simulink model "case9"  (R2024b)
settings: Solver=FixedStepAuto  StartTime=0  StopTime=1  FixedStep=1e-7  RelTol=1e-3
values from neighbouring files (symbols this model uses):
  SG_D_1_D = 0.01056    [IEEE9_case_parameters.m]    (also in case1_parameters.m; case2_parameters.m; case3_parameters.m; case4_parameters.m)
  SG_D_1_EnableSaturation = 0    [IEEE9_case_parameters.m]    (also in case1_parameters.m; case2_parameters.m; case3_parameters.m; case4_parameters.m)
  SG_D_1_f0 = 60    [IEEE9_case_parameters.m]    (also in case1_parameters.m; case2_parameters.m; case3_parameters.m; case4_parameters.m)
  SG_D_1_H = 7.5    [IEEE9_case_parameters.m]    (also in case1_parameters.m; case2_parameters.m; case3_parameters.m; case4_parameters.m)
  SG_D_1_K_A = 20    [IEEE9_case_parameters.m]    (also in case1_parameters.m; case2_parameters.m; case3_parameters.m; case4_parameters.m)
  SG_D_1_K_E = 1.000000e+1    (= 10)    [IEEE9_case_parameters.m]    (also in case1_parameters.m; case2_parameters.m; case3_parameters.m; case4_parameters.m)
  SG_D_1_K_F = 2.363    [IEEE9_case_parameters.m]    (also in case1_parameters.m; case2_parameters.m; case3_parameters.m; case4_parameters.m)
  SG_D_1_K_s = 0.5    [IEEE9_case_parameters.m]    (also in case1_parameters.m = 5; case2_parameters.m = 5; case3_parameters.m = 5; case4_parameters.m = 5)
  SG_D_1_R_a = 0.001088    [IEEE9_case_parameters.m]    (also in case1_parameters.m; case2_parameters.m; case3_parameters.m; case4_parameters.m)
  SG_D_1_S_A = 1    [IEEE9_case_parameters.m]    (also in case1_parameters.m; case2_parameters.m; case3_parameters.m; case4_parameters.m)
  SG_D_1_S_B = 0.103    [IEEE9_case_parameters.m]    (also in case1_parameters.m; case2_parameters.m; case3_parameters.m; case4_parameters.m)
  SG_D_1_S_N = 10.659857    [IEEE9_case_parameters.m]    (also in case1_parameters.m; case2_parameters.m; case3_parameters.m; case4_parameters.m)
  SG_D_1_SpeedPara = 200    [IEEE9_case_parameters.m]    (also in case1_parameters.m; case2_parameters.m; case3_parameters.m; case4_parameters.m)
  SG_D_1_T_0 = 0.720173    [IEEE9_case_parameters.m]    (also in case1_parameters.m = 0.755522; case2_parameters.m = 0.808931; case3_parameters.m = 0.869402; case4_parameters.m = 0.729316)
  SG_D_1_T_1 = 0.3    [IEEE9_case_parameters.m]    (also in case1_parameters.m; case2_parameters.m; case3_parameters.m; case4_parameters.m)
  SG_D_1_T_2 = 0.05    [IEEE9_case_parameters.m]    (also in case1_parameters.m; case2_parameters.m; case3_parameters.m; case4_parameters.m)
  SG_D_1_T_3 = 0.02    [IEEE9_case_parameters.m]    (also in case1_parameters.m; case2_parameters.m; case3_parameters.m; case4_parameters.m)
  SG_D_1_T_4 = 0.005    [IEEE9_case_parameters.m]    (also in case1_parameters.m; case2_parameters.m; case3_parameters.m; case4_parameters.m)
  SG_D_1_T_A = 0.02    [IEEE9_case_parameters.m]    (also in case1_parameters.m; case2_parameters.m; case3_parameters.m; case4_parameters.m)
  SG_D_1_T_dd = 8.000000e+0    (= 8)    [IEEE9_case_parameters.m]    (also in case1_parameters.m; case2_parameters.m; case3_parameters.m; case4_parameters.m)
  SG_D_1_T_ddd = 0.04    [IEEE9_case_parameters.m]    (also in case1_parameters.m; case2_parameters.m; case3_parameters.m; case4_parameters.m)
  SG_D_1_T_E = 0.314    [IEEE9_case_parameters.m]    (also in case1_parameters.m; case2_parameters.m; case3_parameters.m; case4_parameters.m)
  SG_D_1_T_F = 0.35    [IEEE9_case_parameters.m]    (also in case1_parameters.m; case2_parameters.m; case3_parameters.m; case4_parameters.m)
  SG_D_1_T_qd = 0.8    [IEEE9_case_parameters.m]    (also in case1_parameters.m; case2_parameters.m; case3_parameters.m; case4_parameters.m)
  SG_D_1_T_qdd = 0.02    [IEEE9_case_parameters.m]    (also in case1_parameters.m; case2_parameters.m; case3_parameters.m; case4_parameters.m)
  SG_D_1_T_speed = 0.1    [IEEE9_case_parameters.m]    (also in case1_parameters.m = 200; case2_parameters.m = 200; case3_parameters.m = 200; case4_parameters.m = 200)
  SG_D_1_T_w = 0.5    [IEEE9_case_parameters.m]    (also in case1_parameters.m; case2_parameters.m; case3_parameters.m; case4_parameters.m)
  SG_D_1_V_ref = 1.990276    [IEEE9_case_parameters.m]    (also in case1_parameters.m = 2.042296; case2_parameters.m = 2.051388; case3_parameters.m = 2.089584; case4_parameters.m = 2.01845)
  SG_D_1_w_ref = 376.991118    [IEEE9_case_parameters.m]    (also in case1_parameters.m; case2_parameters.m; case3_parameters.m; case4_parameters.m)
  SG_D_1_wb = 6.000000e+1    (= 60)    [IEEE9_case_parameters.m]    (also in case1_parameters.m; case2_parameters.m; case3_parameters.m; case4_parameters.m)
  SG_D_1_x_d = 1.9    [IEEE9_case_parameters.m]    (also in case1_parameters.m; case2_parameters.m; case3_parameters.m; case4_parameters.m)
  SG_D_1_x_dd = 0.302    [IEEE9_case_parameters.m]    (also in case1_parameters.m; case2_parameters.m; case3_parameters.m; case4_parameters.m)
  SG_D_1_x_ddd = 0.204    [IEEE9_case_parameters.m]    (also in case1_parameters.m; case2_parameters.m; case3_parameters.m; case4_parameters.m)
  SG_D_1_x_l = 0.05    [IEEE9_case_parameters.m]    (also in case1_parameters.m; case2_parameters.m; case3_parameters.m; case4_parameters.m)
  SG_D_1_x_q = 1.3    [IEEE9_case_parameters.m]    (also in case1_parameters.m; case2_parameters.m; case3_parameters.m; case4_parameters.m)
  SG_D_1_x_qd = 0.5    [IEEE9_case_parameters.m]    (also in case1_parameters.m; case2_parameters.m; case3_parameters.m; case4_parameters.m)
  SG_D_1_x_qdd = 0.3    [IEEE9_case_parameters.m]    (also in case1_parameters.m; case2_parameters.m; case3_parameters.m; case4_parameters.m)
  SG_D_2_D = 0.02    [IEEE9_case_parameters.m]    (also in case1_parameters.m; case2_parameters.m; case3_parameters.m; case4_parameters.m)
  SG_D_2_EnableSaturation = 0    [IEEE9_case_parameters.m]    (also in case1_parameters.m; case2_parameters.m; case3_parameters.m; case4_parameters.m)
  SG_D_2_f0 = 60    [IEEE9_case_parameters.m]    (also in case1_parameters.m; case2_parameters.m; case3_parameters.m; case4_parameters.m)
  SG_D_2_H = 8.000000e+0    (= 8)    [IEEE9_case_parameters.m]    (also in case1_parameters.m; case2_parameters.m; case3_parameters.m; case4_parameters.m)
  SG_D_2_K_A = 20    [IEEE9_case_parameters.m]    (also in case1_parameters.m; case2_parameters.m; case3_parameters.m; case4_parameters.m)
  SG_D_2_K_E = 1.000000e+1    (= 10)    [IEEE9_case_parameters.m]    (also in case1_parameters.m; case2_parameters.m; case3_parameters.m; case4_parameters.m)
  SG_D_2_K_F = 2.363    [IEEE9_case_parameters.m]    (also in case1_parameters.m; case2_parameters.m; case3_parameters.m; case4_parameters.m)
  SG_D_2_K_s = 0.5    [IEEE9_case_parameters.m]    (also in case1_parameters.m = 4; case2_parameters.m = 4; case3_parameters.m = 4; case4_parameters.m = 4)
  SG_D_2_R_a = 0.001088    [IEEE9_case_parameters.m]    (also in case1_parameters.m; case2_parameters.m; case3_parameters.m; case4_parameters.m)
  SG_D_2_S_A = 1    [IEEE9_case_parameters.m]    (also in case1_parameters.m; case2_parameters.m; case3_parameters.m; case4_parameters.m)
  SG_D_2_S_B = 0.103    [IEEE9_case_parameters.m]    (also in case1_parameters.m; case2_parameters.m; case3_parameters.m; case4_parameters.m)
  SG_D_2_S_N = 10.659857    [IEEE9_case_parameters.m]    (also in case1_parameters.m; case2_parameters.m; case3_parameters.m; case4_parameters.m)
  SG_D_2_SpeedPara = 200    [IEEE9_case_parameters.m]    (also in case1_parameters.m; case2_parameters.m; case3_parameters.m; case4_parameters.m)
  SG_D_2_T_0 = 1.632913    [IEEE9_case_parameters.m]    (also in case1_parameters.m = 1.632925; case2_parameters.m = 1.632915; case3_parameters.m = 1.632914; case4_parameters.m = 1.632927)
  SG_D_2_T_1 = 0.2    [IEEE9_case_parameters.m]    (also in case1_parameters.m; case2_parameters.m; case3_parameters.m; case4_parameters.m)
  SG_D_2_T_2 = 0.05    [IEEE9_case_parameters.m]    (also in case1_parameters.m; case2_parameters.m; case3_parameters.m; case4_parameters.m)
  SG_D_2_T_3 = 0.02    [IEEE9_case_parameters.m]    (also in case1_parameters.m; case2_parameters.m; case3_parameters.m; case4_parameters.m)
  SG_D_2_T_4 = 0.005    [IEEE9_case_parameters.m]    (also in case1_parameters.m; case2_parameters.m; case3_parameters.m; case4_parameters.m)
  SG_D_2_T_A = 0.02    [IEEE9_case_parameters.m]    (also in case1_parameters.m; case2_parameters.m; case3_parameters.m; case4_parameters.m)
  SG_D_2_T_dd = 7.9    [IEEE9_case_parameters.m]    (also in case1_parameters.m; case2_parameters.m; case3_parameters.m; case4_parameters.m)
  SG_D_2_T_ddd = 0.04    [IEEE9_case_parameters.m]    (also in case1_parameters.m; case2_parameters.m; case3_parameters.m; case4_parameters.m)
  SG_D_2_T_E = 0.314    [IEEE9_case_parameters.m]    (also in case1_parameters.m; case2_parameters.m; case3_parameters.m; case4_parameters.m)
  SG_D_2_T_F = 0.35    [IEEE9_case_parameters.m]    (also in case1_parameters.m; case2_parameters.m; case3_parameters.m; case4_parameters.m)
  SG_D_2_T_qd = 0.8    [IEEE9_case_parameters.m]    (also in case1_parameters.m; case2_parameters.m; case3_parameters.m; case4_parameters.m)
  SG_D_2_T_qdd = 0.015    [IEEE9_case_parameters.m]    (also in case1_parameters.m; case2_parameters.m; case3_parameters.m; case4_parameters.m)
  SG_D_2_T_speed = 0.1    [IEEE9_case_parameters.m]    (also in case1_parameters.m = 150; case2_parameters.m = 150; case3_parameters.m = 150; case4_parameters.m = 150)
  SG_D_2_T_w = 0.35    [IEEE9_case_parameters.m]    (also in case1_parameters.m; case2_parameters.m; case3_parameters.m; case4_parameters.m)
  SG_D_2_V_ref = 2.58547    [IEEE9_case_parameters.m]    (also in case1_parameters.m = 2.597896; case2_parameters.m = 2.587136; case3_parameters.m = 2.586042; case4_parameters.m = 2.599679)
  SG_D_2_w_ref = 376.991118    [IEEE9_case_parameters.m]    (also in case1_parameters.m; case2_parameters.m; case3_parameters.m; case4_parameters.m)
  SG_D_2_wb = 6.000000e+1    (= 60)    [IEEE9_case_parameters.m]    (also in case1_parameters.m; case2_parameters.m; case3_parameters.m; case4_parameters.m)
  SG_D_2_x_d = 1.8    [IEEE9_case_parameters.m]    (also in case1_parameters.m; case2_parameters.m; case3_parameters.m; case4_parameters.m)
  SG_D_2_x_dd = 0.302    [IEEE9_case_parameters.m]    (also in case1_parameters.m; case2_parameters.m; case3_parameters.m; case4_parameters.m)
  SG_D_2_x_ddd = 0.204    [IEEE9_case_parameters.m]    (also in case1_parameters.m; case2_parameters.m; case3_parameters.m; case4_parameters.m)
  SG_D_2_x_l = 0.05    [IEEE9_case_parameters.m]    (also in case1_parameters.m; case2_parameters.m; case3_parameters.m; case4_parameters.m)
  SG_D_2_x_q = 1.25    [IEEE9_case_parameters.m]    (also in case1_parameters.m; case2_parameters.m; case3_parameters.m; case4_parameters.m)
  SG_D_2_x_qd = 0.5    [IEEE9_case_parameters.m]    (also in case1_parameters.m; case2_parameters.m; case3_parameters.m; case4_parameters.m)
  SG_D_2_x_qdd = 0.3    [IEEE9_case_parameters.m]    (also in case1_parameters.m; case2_parameters.m; case3_parameters.m; case4_parameters.m)
  SG_D_3_D = 0.02    [IEEE9_case_parameters.m]    (also in case1_parameters.m; case2_parameters.m; case3_parameters.m; case4_parameters.m)
  SG_D_3_EnableSaturation = 0    [IEEE9_case_parameters.m]    (also in case1_parameters.m; case2_parameters.m; case3_parameters.m; case4_parameters.m)
  SG_D_3_f0 = 60    [IEEE9_case_parameters.m]    (also in case1_parameters.m; case2_parameters.m; case3_parameters.m; case4_parameters.m)
  SG_D_3_H = 7.7    [IEEE9_case_parameters.m]    (also in case1_parameters.m; case2_parameters.m; case3_parameters.m; case4_parameters.m)
  SG_D_3_K_A = 20    [IEEE9_case_parameters.m]    (also in case1_parameters.m; case2_parameters.m; case3_parameters.m; case4_parameters.m)
  SG_D_3_K_E = 1.000000e+1    (= 10)    [IEEE9_case_parameters.m]    (also in case1_parameters.m; case2_parameters.m; case3_parameters.m; case4_parameters.m)
  SG_D_3_K_F = 2.363    [IEEE9_case_parameters.m]    (also in case1_parameters.m; case2_parameters.m; case3_parameters.m; case4_parameters.m)
  SG_D_3_K_s = 0.2    [IEEE9_case_parameters.m]    (also in case1_parameters.m = 2; case2_parameters.m = 2; case3_parameters.m = 2; case4_parameters.m = 2)
  SG_D_3_R_a = 0.001088    [IEEE9_case_parameters.m]    (also in case1_parameters.m; case2_parameters.m; case3_parameters.m; case4_parameters.m)
  SG_D_3_S_A = 1    [IEEE9_case_parameters.m]    (also in case1_parameters.m; case2_parameters.m; case3_parameters.m; case4_parameters.m)
  SG_D_3_S_B = 0.103    [IEEE9_case_parameters.m]    (also in case1_parameters.m; case2_parameters.m; case3_parameters.m; case4_parameters.m)
  SG_D_3_S_N = 10.659857    [IEEE9_case_parameters.m]    (also in case1_parameters.m; case2_parameters.m; case3_parameters.m; case4_parameters.m)
  SG_D_3_SpeedPara = 200    [IEEE9_case_parameters.m]    (also in case1_parameters.m; case2_parameters.m; case3_parameters.m; case4_parameters.m)
  SG_D_3_T_0 = 0.850788    [IEEE9_case_parameters.m]    (also in case1_parameters.m = 0.850786; case2_parameters.m = 0.850787; case3_parameters.m; case4_parameters.m = 0.850786)
  SG_D_3_T_1 = 0.2    [IEEE9_case_parameters.m]    (also in case1_parameters.m; case2_parameters.m; case3_parameters.m; case4_parameters.m)
  SG_D_3_T_2 = 0.05    [IEEE9_case_parameters.m]    (also in case1_parameters.m; case2_parameters.m; case3_parameters.m; case4_parameters.m)
  SG_D_3_T_3 = 0.02    [IEEE9_case_parameters.m]    (also in case1_parameters.m; case2_parameters.m; case3_parameters.m; case4_parameters.m)
  SG_D_3_T_4 = 0.005    [IEEE9_case_parameters.m]    (also in case1_parameters.m; case2_parameters.m; case3_parameters.m; case4_parameters.m)
  SG_D_3_T_A = 0.02    [IEEE9_case_parameters.m]    (also in case1_parameters.m; case2_parameters.m; case3_parameters.m; case4_parameters.m)
  SG_D_3_T_dd = 8.1    [IEEE9_case_parameters.m]    (also in case1_parameters.m; case2_parameters.m; case3_parameters.m; case4_parameters.m)
  SG_D_3_T_ddd = 0.04    [IEEE9_case_parameters.m]    (also in case1_parameters.m; case2_parameters.m; case3_parameters.m; case4_parameters.m)
  SG_D_3_T_E = 0.314    [IEEE9_case_parameters.m]    (also in case1_parameters.m; case2_parameters.m; case3_parameters.m; case4_parameters.m)
  SG_D_3_T_F = 0.35    [IEEE9_case_parameters.m]    (also in case1_parameters.m; case2_parameters.m; case3_parameters.m; case4_parameters.m)
  SG_D_3_T_qd = 0.8    [IEEE9_case_parameters.m]    (also in case1_parameters.m; case2_parameters.m; case3_parameters.m; case4_parameters.m)
  SG_D_3_T_qdd = 0.015    [IEEE9_case_parameters.m]    (also in case1_parameters.m; case2_parameters.m; case3_parameters.m; case4_parameters.m)
  SG_D_3_T_speed = 0.1    [IEEE9_case_parameters.m]    (also in case1_parameters.m = 180; case2_parameters.m = 180; case3_parameters.m = 180; case4_parameters.m = 180)
  SG_D_3_T_w = 0.4    [IEEE9_case_parameters.m]    (also in case1_parameters.m; case2_parameters.m; case3_parameters.m; case4_parameters.m)
  SG_D_3_V_ref = 1.892727    [IEEE9_case_parameters.m]    (also in case1_parameters.m = 1.906439; case2_parameters.m = 1.895535; case3_parameters.m = 1.892105; case4_parameters.m = 1.906598)
  SG_D_3_w_ref = 376.991118    [IEEE9_case_parameters.m]    (also in case1_parameters.m; case2_parameters.m; case3_parameters.m; case4_parameters.m)
  SG_D_3_wb = 6.000000e+1    (= 60)    [IEEE9_case_parameters.m]    (also in case1_parameters.m; case2_parameters.m; case3_parameters.m; case4_parameters.m)
  SG_D_3_x_d = 1.85    [IEEE9_case_parameters.m]    (also in case1_parameters.m; case2_parameters.m; case3_parameters.m; case4_parameters.m)
  SG_D_3_x_dd = 0.302    [IEEE9_case_parameters.m]    (also in case1_parameters.m; case2_parameters.m; case3_parameters.m; case4_parameters.m)
  SG_D_3_x_ddd = 0.204    [IEEE9_case_parameters.m]    (also in case1_parameters.m; case2_parameters.m; case3_parameters.m; case4_parameters.m)
  SG_D_3_x_l = 0.05    [IEEE9_case_parameters.m]    (also in case1_parameters.m; case2_parameters.m; case3_parameters.m; case4_parameters.m)
  SG_D_3_x_q = 1.2    [IEEE9_case_parameters.m]    (also in case1_parameters.m; case2_parameters.m; case3_parameters.m; case4_parameters.m)
  SG_D_3_x_qd = 0.5    [IEEE9_case_parameters.m]    (also in case1_parameters.m; case2_parameters.m; case3_parameters.m; case4_parameters.m)
  SG_D_3_x_qdd = 0.3    [IEEE9_case_parameters.m]    (also in case1_parameters.m; case2_parameters.m; case3_parameters.m; case4_parameters.m)
(part 5 of 12)

== system case9/Apparatus/SG_D_1/d_T_m_SG_D_1_block ==
  note: d_T_m_SG_D_1 in case9
      | $-\frac{T_{m,\mathrm{SG},D,1}-T_{0}+\frac{\mathrm{SpeedPara}\,\left(w_{\mathrm{SG},D,1}-w_{\mathrm{ref}}\right)}{2\,f_{0}\,\pi }}{T_{\mathrm{speed}}}$
      | Automatically generated on 2025-10-31 19:34:43 .
  State_w_SG_D_1_70e26 : Inport
  State_T_m_SG_D_1_20e91 : Inport  Port=2
  Add_0d769 : Sum
  Add_b171e : Sum
  Constant_-1_adbd7 : Constant  Value=-1
  Constant_2.0_9a548 : Constant  Value=2.0
  Constant_SpeedPara_b6f64 : Constant  Value=SpeedPara
  Constant_T_0_27b37 : Constant  Value=T_0
  Constant_T_speed_09f5e : Constant  Value=T_speed
  Constant_f0_5920a : Constant  Value=f0
  Constant_pi_1982f : Constant  Value=pi
  Constant_w_ref_24065 : Constant  Value=w_ref
  Divide_b205f : Product  Inputs=*/
  Divide_dc274 : Product  Inputs=*/
  Product_2da8b : Product
  Product_66494 : Product
  Product_92c7a : Product
  Product_bb807 : Product
  Subtract_8dfc6 : Sum  Inputs=+-
  Blockout_d_T_m_SG_D_1_fd2e1 : Outport
  wires:
  Constant_-1_adbd7/1 -> Product_92c7a/1
  Constant_w_ref_24065/1 -> Add_b171e/2
  State_w_SG_D_1_70e26/1 -> Product_92c7a/2
  Add_0d769/1 -> Subtract_8dfc6/1
  Add_b171e/1 -> Product_bb807/2
  Product_92c7a/1 -> Add_b171e/1
  Constant_2.0_9a548/1 -> Product_66494/1
  Constant_pi_1982f/1 -> Product_66494/2
  Constant_SpeedPara_b6f64/1 -> Product_bb807/1
  Product_66494/1 -> Product_2da8b/1
  Constant_f0_5920a/1 -> Product_2da8b/2
  Constant_T_speed_09f5e/1 -> Divide_dc274/2
  Product_bb807/1 -> Divide_b205f/1
  Product_2da8b/1 -> Divide_b205f/2
  Divide_b205f/1 -> Add_0d769/1
  Constant_T_0_27b37/1 -> Add_0d769/2
  State_T_m_SG_D_1_20e91/1 -> Subtract_8dfc6/2
  Subtract_8dfc6/1 -> Divide_dc274/1
  Divide_dc274/1 -> Blockout_d_T_m_SG_D_1_fd2e1/1

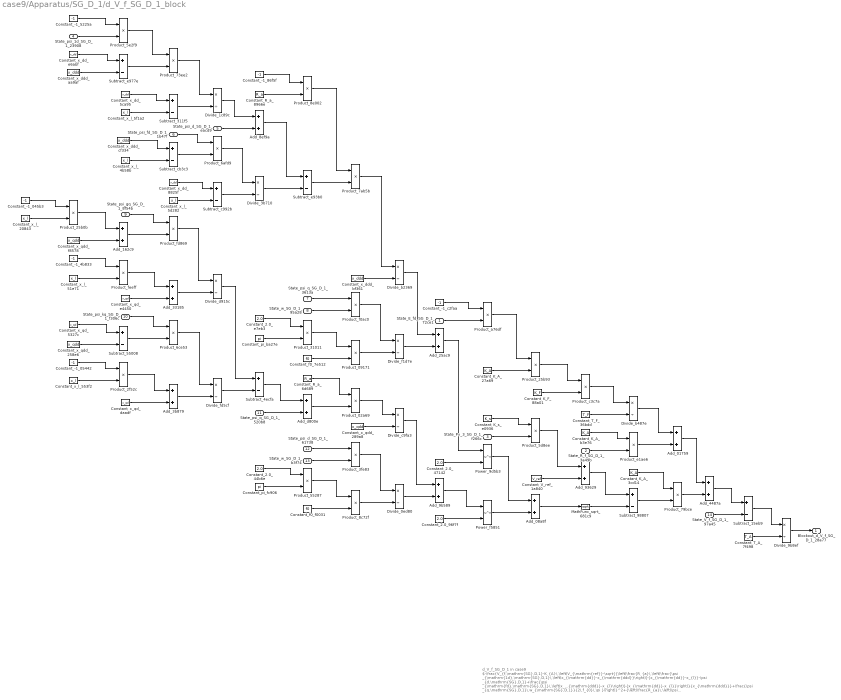
== system case9/Apparatus/SG_D_1/d_V_f_SG_D_1_block ==
  note: d_V_f_SG_D_1 in case9
      | $-\frac{V_{f,\mathrm{SG},D,1}-K_{A}\,\left(V_{\mathrm{ref}}-\sqrt{{\left(\frac{R_{a}\,\left(\frac{\psi _{\mathrm{1d},\mathrm{SG},D,1}\,\left(x_{\mathrm{dd}}-x_{\mathrm{ddd}}\right)}{x_{\mathrm{dd}}-x_{l}}-\psi _{d,\mathrm{SG},D,1}+\frac{\psi _{\mathrm{fd},\mathrm{SG},D,1}\,\left(x_{\mathrm{ddd}}-x_{l}\right)}{x_{\mathrm{dd}}-x_{l}}\right)}{x_{\mathrm{ddd}}}+\frac{\psi _{q,\mathrm{SG},D,1}\,w_{\mathrm{SG},D,1}}{2\,f_{0}\,\pi }\right)}^2+{\left(\frac{R_{a}\,\left(\psi _{q,\mathrm{SG},D,1}+\frac{\psi _{\mathrm{gq},\mathrm{SG},D,1}\,\left(x_{l}-x_{\mathrm{qdd}}\right)}{x_{l}-x_{\mathrm{qd}}}+\frac{\psi _{\mathrm{kq},\mathrm{SG},D,1}\,\left(x_{\mathrm{qd}}-x_{\mathrm{qdd}}\right)}{x_{l}-x_{\mathrm{qd}}}\right)}{x_{\mathrm{qdd}}}+\frac{\psi _{d,\mathrm{SG},D,1}\,w_{\mathrm{SG},D,1}}{2\,f_{0}\,\pi }\right)}^2}+K_{s}\,\mathrm{Px}_{3,\mathrm{SG},D,1}\right)-K_{A}\,R_{f,\mathrm{SG},D,1}+\frac{E_{\mathrm{fd},\mathrm{SG},D,1}\,K_{A}\,K_{F}}{T_{F}}}{T_{A}}$
      | Automatically generated on 2025-10-31 19:34:45 .
  State_E_fd_SG_D_1_72ce1 : Inport
  State_R_f_SG_D_1_3a49b : Inport  Port=2
  State_Px_3_SG_D_1_f266c : Inport  Port=3
  State_psi_1d_SG_D_1_23908 : Inport  Port=4
  State_psi_d_SG_D_1_eacd9 : Inport  Port=5
  State_psi_fd_SG_D_1_1b47f : Inport  Port=6
  State_psi_q_SG_D_1_3613a : Inport  Port=7
  State_w_SG_D_1_95a28 : Inport  Port=8
  State_psi_gq_SG_D_1_8f54b : Inport  Port=9
  State_psi_kq_SG_D_1_f306c : Inport  Port=10
  State_psi_q_SG_D_1_520b8 : Inport  Port=11
  State_psi_d_SG_D_1_61738 : Inport  Port=12
  State_w_SG_D_1_b3f74 : Inport  Port=13
  State_V_f_SG_D_1_97a45 : Inport  Port=14
  Add_01759 : Sum
  Add_08a8f : Sum
  Add_162c9 : Sum
  Add_25ac9 : Sum
  Add_33185 : Sum
  Add_3b879 : Sum
  Add_4487a : Sum
  Add_8ef9a : Sum
  Add_93629 : Sum
  Add_9b589 : Sum
  Add_d800e : Sum
  Constant_-1_045b3 : Constant  Value=-1
  Constant_-1_05442 : Constant  Value=-1
  Constant_-1_4b833 : Constant  Value=-1
  Constant_-1_5225a : Constant  Value=-1
  Constant_-1_86f5f : Constant  Value=-1
  Constant_-1_c2faa : Constant  Value=-1
  Constant_2.0_44b6e : Constant  Value=2.0
  Constant_2.0_47142 : Constant  Value=2.0
  Constant_2.0_96f7f : Constant  Value=2.0
  Constant_2.0_e7eb3 : Constant  Value=2.0
  Constant_K_A_27a69 : Constant  Value=K_A
  Constant_K_A_3cd14 : Constant  Value=K_A
  Constant_K_A_b3e76 : Constant  Value=K_A
  Constant_K_F_88a01 : Constant  Value=K_F
  Constant_K_s_e0936 : Constant  Value=K_s
  Constant_R_a_6d689 : Constant  Value=R_a
  Constant_R_a_8966e : Constant  Value=R_a
  Constant_T_A_7f498 : Constant  Value=T_A
  Constant_T_F_36bdd : Constant  Value=T_F
  Constant_V_ref_1a840 : Constant  Value=V_ref
  Constant_f0_7e512 : Constant  Value=f0
  Constant_f0_f0031 : Constant  Value=f0
  Constant_pi_ba27e : Constant  Value=pi
  Constant_pi_fc906 : Constant  Value=pi
  Constant_x_dd_5ca95 : Constant  Value=x_dd
  Constant_x_dd_8825f : Constant  Value=x_dd
  Constant_x_dd_e6abf : Constant  Value=x_dd
  Constant_x_ddd_aa9af : Constant  Value=x_ddd
  Constant_x_ddd_bf361 : Constant  Value=x_ddd
  Constant_x_ddd_cf334 : Constant  Value=x_ddd
  Constant_x_l_20843 : Constant  Value=x_l
  Constant_x_l_4b58b : Constant  Value=x_l
  Constant_x_l_51e71 : Constant  Value=x_l
  Constant_x_l_553f2 : Constant  Value=x_l
  Constant_x_l_5d282 : Constant  Value=x_l
  Constant_x_l_5f1a2 : Constant  Value=x_l
  Constant_x_qd_5327c : Constant  Value=x_qd
  Constant_x_qd_daadf : Constant  Value=x_qd
  Constant_x_qd_e4450 : Constant  Value=x_qd
  Constant_x_qdd_258e6 : Constant  Value=x_qdd
  Constant_x_qdd_289a8 : Constant  Value=x_qdd
  Constant_x_qdd_f8578 : Constant  Value=x_qdd
  Divide_0ed80 : Product  Inputs=*/
  Divide_1c89c : Product  Inputs=*/
  Divide_3b710 : Product  Inputs=*/
  Divide_9b8ef : Product  Inputs=*/
  Divide_b2369 : Product  Inputs=*/
  Divide_b487e : Product  Inputs=*/
  Divide_c9fa3 : Product  Inputs=*/
  Divide_d915c : Product  Inputs=*/
  Divide_f1d7e : Product  Inputs=*/
  Divide_fd5cf : Product  Inputs=*/
  MathFunc_sqrt_681c9 : Sqrt
  Power_9d5b3 : Math  Operator=pow
  Power_f5851 : Math  Operator=pow
  Product_02a69 : Product
  Product_09171 : Product
  Product_25b0b : Product
  Product_25b93 : Product
  Product_2f52c : Product
  Product_31011 : Product
  Product_3fe83 : Product
  Product_55287 : Product
  Product_5d8ee : Product
  Product_5e2f9 : Product
  Product_6afd9 : Product
  Product_6ce53 : Product
  Product_73ee2 : Product
  Product_79bce : Product
  Product_7ab5b : Product
  Product_8c72f : Product
  Product_8e002 : Product
  Product_a76df : Product
  Product_c3c7a : Product
  Product_e1ae6 : Product
  Product_f0ac0 : Product
  Product_fd869 : Product
  Product_feeff : Product
  Subtract_15eb9 : Sum  Inputs=+-
  Subtract_311f5 : Sum  Inputs=+-
  Subtract_4ecfa : Sum  Inputs=+-
  Subtract_55008 : Sum  Inputs=+-
  Subtract_98807 : Sum  Inputs=+-
  Subtract_c992b : Sum  Inputs=+-
  Subtract_cb3c3 : Sum  Inputs=+-
  Subtract_e93b0 : Sum  Inputs=+-
  Subtract_e977e : Sum  Inputs=+-
  Blockout_d_V_f_SG_D_1_28a77 : Outport
  wires:
  Constant_-1_05442/1 -> Product_2f52c/1
  Constant_-1_045b3/1 -> Product_25b0b/1
  State_psi_d_SG_D_1_61738/1 -> Product_3fe83/1
  Constant_x_qd_daadf/1 -> Add_3b879/2
  Constant_x_qdd_f8578/1 -> Add_162c9/2
  State_w_SG_D_1_b3f74/1 -> Product_3fe83/2
  Constant_x_l_20843/1 -> Product_25b0b/2
  Subtract_e93b0/1 -> Product_7ab5b/2
  Constant_x_l_553f2/1 -> Product_2f52c/2
  Constant_x_dd_e6abf/1 -> Subtract_e977e/1
  Constant_R_a_8966e/1 -> Product_8e002/2
  Constant_-1_5225a/1 -> Product_5e2f9/1
  Divide_3b710/1 -> Subtract_e93b0/2
  Constant_x_ddd_aa9af/1 -> Subtract_e977e/2
  Add_3b879/1 -> Divide_fd5cf/2
  State_psi_1d_SG_D_1_23908/1 -> Product_5e2f9/2
  Add_33185/1 -> Divide_d915c/2
  Subtract_55008/1 -> Product_6ce53/2
  Product_c3c7a/1 -> Divide_b487e/1
  Product_31011/1 -> Product_09171/1
  Product_25b0b/1 -> Add_162c9/1
  Constant_-1_4b833/1 -> Product_feeff/1
  Constant_x_l_51e71/1 -> Product_feeff/2
  Add_8ef9a/1 -> Subtract_e93b0/1
  Constant_2.0_44b6e/1 -> Product_55287/1
  Constant_x_qd_5327c/1 -> Subtract_55008/1
  Product_5e2f9/1 -> Product_73ee2/1
  Constant_pi_fc906/1 -> Product_55287/2
  Constant_x_qdd_258e6/1 -> Subtract_55008/2
  Subtract_e977e/1 -> Product_73ee2/2
  State_psi_q_SG_D_1_520b8/1 -> Add_d800e/2
  Constant_x_dd_5ca95/1 -> Subtract_311f5/1
  Constant_x_l_5f1a2/1 -> Subtract_311f5/2
  Constant_x_ddd_cf334/1 -> Subtract_cb3c3/1
  Constant_x_l_4b58b/1 -> Subtract_cb3c3/2
  State_psi_gq_SG_D_1_8f54b/1 -> Product_fd869/1
  Add_162c9/1 -> Product_fd869/2
  Product_feeff/1 -> Add_33185/1
  Constant_x_qd_e4450/1 -> Add_33185/2
  Divide_1c89c/1 -> Add_8ef9a/1
  Subtract_311f5/1 -> Divide_1c89c/2
  State_psi_kq_SG_D_1_f306c/1 -> Product_6ce53/1
  Divide_9b8ef/1 -> Blockout_d_V_f_SG_D_1_28a77/1
  Product_2f52c/1 -> Add_3b879/1
  Product_73ee2/1 -> Divide_1c89c/1
  State_psi_fd_SG_D_1_1b47f/1 -> Product_6afd9/1
  State_w_SG_D_1_95a28/1 -> Product_f0ac0/2
  Subtract_cb3c3/1 -> Product_6afd9/2
  Constant_x_dd_8825f/1 -> Subtract_c992b/1
  Constant_x_l_5d282/1 -> Subtract_c992b/2
  Product_fd869/1 -> Divide_d915c/1
  Product_8e002/1 -> Product_7ab5b/1
  Product_6ce53/1 -> Divide_fd5cf/1
  State_psi_d_SG_D_1_eacd9/1 -> Add_8ef9a/2
  Product_6afd9/1 -> Divide_3b710/1
  Subtract_c992b/1 -> Divide_3b710/2
  Divide_d915c/1 -> Subtract_4ecfa/1
  Divide_fd5cf/1 -> Subtract_4ecfa/2
  Constant_-1_86f5f/1 -> Product_8e002/1
  Constant_2.0_e7eb3/1 -> Product_31011/1
  Constant_pi_ba27e/1 -> Product_31011/2
  Subtract_4ecfa/1 -> Add_d800e/1
  State_psi_q_SG_D_1_3613a/1 -> Product_f0ac0/1
  Constant_f0_7e512/1 -> Product_09171/2
  Constant_R_a_6d689/1 -> Product_02a69/1
  Add_d800e/1 -> Product_02a69/2
  Product_55287/1 -> Product_8c72f/1
  Power_9d5b3/1 -> Add_08a8f/1
  Constant_f0_f0031/1 -> Product_8c72f/2
  Product_7ab5b/1 -> Divide_b2369/1
  Constant_x_ddd_bf361/1 -> Divide_b2369/2
  Product_f0ac0/1 -> Divide_f1d7e/1
  Product_09171/1 -> Divide_f1d7e/2
  Product_02a69/1 -> Divide_c9fa3/1
  Constant_x_qdd_289a8/1 -> Divide_c9fa3/2
  Product_3fe83/1 -> Divide_0ed80/1
  Product_8c72f/1 -> Divide_0ed80/2
  Divide_b2369/1 -> Add_25ac9/1
  Divide_f1d7e/1 -> Add_25ac9/2
  Divide_c9fa3/1 -> Add_9b589/1
  Divide_0ed80/1 -> Add_9b589/2
  Constant_-1_c2faa/1 -> Product_a76df/1
  State_E_fd_SG_D_1_72ce1/1 -> Product_a76df/2
  Add_25ac9/1 -> Power_9d5b3/1
  Constant_2.0_47142/1 -> Power_9d5b3/2
  Add_9b589/1 -> Power_f5851/1
  Constant_2.0_96f7f/1 -> Power_f5851/2
  Product_a76df/1 -> Product_25b93/1
  Constant_K_A_27a69/1 -> Product_25b93/2
  Constant_K_s_e0936/1 -> Product_5d8ee/1
  State_Px_3_SG_D_1_f266c/1 -> Product_5d8ee/2
  Power_f5851/1 -> Add_08a8f/2
  Divide_b487e/1 -> Add_01759/1
  Product_25b93/1 -> Product_c3c7a/1
  Constant_K_F_88a01/1 -> Product_c3c7a/2
  Product_5d8ee/1 -> Add_93629/1
  Constant_V_ref_1a840/1 -> Add_93629/2
  Add_08a8f/1 -> MathFunc_sqrt_681c9/1
  Constant_T_F_36bdd/1 -> Divide_b487e/2
  Constant_K_A_b3e76/1 -> Product_e1ae6/1
  State_R_f_SG_D_1_3a49b/1 -> Product_e1ae6/2
  Add_93629/1 -> Subtract_98807/1
  MathFunc_sqrt_681c9/1 -> Subtract_98807/2
  Constant_T_A_7f498/1 -> Divide_9b8ef/2
  Product_e1ae6/1 -> Add_01759/2
  Constant_K_A_3cd14/1 -> Product_79bce/1
  Subtract_98807/1 -> Product_79bce/2
  Add_01759/1 -> Add_4487a/1
  Product_79bce/1 -> Add_4487a/2
  Add_4487a/1 -> Subtract_15eb9/1
  State_V_f_SG_D_1_97a45/1 -> Subtract_15eb9/2
  Subtract_15eb9/1 -> Divide_9b8ef/1

== system case9/Apparatus/SG_D_1/d_psi_1d_SG_D_1_block ==
  note: d_psi_1d_SG_D_1 in case9
      | $-\frac{\psi _{\mathrm{1d},\mathrm{SG},D,1}-\psi _{\mathrm{fd},\mathrm{SG},D,1}+\frac{\left(x_{\mathrm{dd}}-x_{l}\right)\,\left(\frac{\psi _{\mathrm{1d},\mathrm{SG},D,1}\,\left(x_{\mathrm{dd}}-x_{\mathrm{ddd}}\right)}{x_{\mathrm{dd}}-x_{l}}-\psi _{d,\mathrm{SG},D,1}+\frac{\psi _{\mathrm{fd},\mathrm{SG},D,1}\,\left(x_{\mathrm{ddd}}-x_{l}\right)}{x_{\mathrm{dd}}-x_{l}}\right)}{x_{\mathrm{ddd}}}}{T_{\mathrm{ddd}}}$
      | Automatically generated on 2025-10-31 19:34:39 .
  State_psi_1d_SG_D_1_47d5b : Inport
  State_psi_fd_SG_D_1_d2d5e : Inport  Port=2
  State_psi_1d_SG_D_1_e9060 : Inport  Port=3
  State_psi_d_SG_D_1_5aef1 : Inport  Port=4
  State_psi_fd_SG_D_1_3a491 : Inport  Port=5
  Add_1b0a4 : Sum
  Add_eb0ff : Sum
  Add_f82a1 : Sum
  Constant_-1_67226 : Constant  Value=-1
  Constant_-1_f7a70 : Constant  Value=-1
  Constant_T_ddd_60904 : Constant  Value=T_ddd
  Constant_x_dd_02615 : Constant  Value=x_dd
  Constant_x_dd_821c7 : Constant  Value=x_dd
  Constant_x_dd_826e0 : Constant  Value=x_dd
  Constant_x_dd_e2833 : Constant  Value=x_dd
  Constant_x_ddd_58068 : Constant  Value=x_ddd
  Constant_x_ddd_69a4a : Constant  Value=x_ddd
  Constant_x_ddd_ad741 : Constant  Value=x_ddd
  Constant_x_l_26a18 : Constant  Value=x_l
  Constant_x_l_2dd4b : Constant  Value=x_l
  Constant_x_l_6f905 : Constant  Value=x_l
  Constant_x_l_92289 : Constant  Value=x_l
  Divide_25ffc : Product  Inputs=*/
  Divide_29beb : Product  Inputs=*/
  Divide_3ba7e : Product  Inputs=*/
  Divide_fd233 : Product  Inputs=*/
  Product_0ada7 : Product
  Product_332db : Product
  Product_668b5 : Product
  Product_fc799 : Product
  Product_fd988 : Product
  Subtract_7f358 : Sum  Inputs=+-
  Subtract_8bdd4 : Sum  Inputs=+-
  Subtract_aa8fc : Sum  Inputs=+-
  Subtract_b2c81 : Sum  Inputs=+-
  Subtract_c7cc3 : Sum  Inputs=+-
  Subtract_db678 : Sum  Inputs=+-
  Blockout_d_psi_1d_SG_D_1_60e48 : Outport
  wires:
  Product_332db/1 -> Product_0ada7/1
  Constant_-1_f7a70/1 -> Product_332db/1
  Subtract_7f358/1 -> Product_0ada7/2
  State_psi_1d_SG_D_1_e9060/1 -> Product_332db/2
  Subtract_b2c81/1 -> Product_fd988/1
  State_psi_d_SG_D_1_5aef1/1 -> Add_f82a1/2
  Constant_x_dd_e2833/1 -> Subtract_8bdd4/1
  Constant_x_l_92289/1 -> Subtract_b2c81/2
  Constant_x_dd_821c7/1 -> Subtract_7f358/1
  Subtract_aa8fc/1 -> Product_fc799/2
  Constant_x_l_26a18/1 -> Subtract_8bdd4/2
  Divide_fd233/1 -> Subtract_c7cc3/2
  Constant_x_ddd_ad741/1 -> Subtract_7f358/2
  Constant_x_ddd_58068/1 -> Subtract_aa8fc/1
  Constant_x_l_2dd4b/1 -> Subtract_aa8fc/2
  Add_1b0a4/1 -> Add_eb0ff/1
  Product_0ada7/1 -> Divide_29beb/1
  Divide_25ffc/1 -> Add_eb0ff/2
  Subtract_8bdd4/1 -> Divide_29beb/2
  State_psi_fd_SG_D_1_3a491/1 -> Product_fc799/1
  Constant_x_dd_02615/1 -> Subtract_db678/1
  Constant_x_l_6f905/1 -> Subtract_db678/2
  Constant_x_ddd_69a4a/1 -> Divide_25ffc/2
  Subtract_c7cc3/1 -> Product_fd988/2
  Divide_29beb/1 -> Add_f82a1/1
  Product_fc799/1 -> Divide_fd233/1
  Subtract_db678/1 -> Divide_fd233/2
  Product_fd988/1 -> Divide_25ffc/1
  Constant_x_dd_826e0/1 -> Subtract_b2c81/1
  Add_f82a1/1 -> Subtract_c7cc3/1
  Constant_-1_67226/1 -> Product_668b5/1
  State_psi_1d_SG_D_1_47d5b/1 -> Product_668b5/2
  Product_668b5/1 -> Add_1b0a4/1
  State_psi_fd_SG_D_1_d2d5e/1 -> Add_1b0a4/2
  Add_eb0ff/1 -> Divide_3ba7e/1
  Constant_T_ddd_60904/1 -> Divide_3ba7e/2
  Divide_3ba7e/1 -> Blockout_d_psi_1d_SG_D_1_60e48/1

== system case9/Apparatus/SG_D_1/d_psi_d_SG_D_1_block ==
  note: d_psi_d_SG_D_1 in case9
      | $2\,\pi \,f_{0}\,\left(v_{d,\mathrm{SG},D,1}\,\sin\left(\theta _{\mathrm{SG},D,1}\right)-v_{q,\mathrm{SG},D,1}\,\cos\left(\theta _{\mathrm{SG},D,1}\right)+\frac{R_{a}\,\left(\frac{\psi _{\mathrm{1d},\mathrm{SG},D,1}\,\left(x_{\mathrm{dd}}-x_{\mathrm{ddd}}\right)}{x_{\mathrm{dd}}-x_{l}}-\psi _{d,\mathrm{SG},D,1}+\frac{\psi _{\mathrm{fd},\mathrm{SG},D,1}\,\left(x_{\mathrm{ddd}}-x_{l}\right)}{x_{\mathrm{dd}}-x_{l}}\right)}{x_{\mathrm{ddd}}}+\frac{\psi _{q,\mathrm{SG},D,1}\,w_{\mathrm{SG},D,1}}{2\,f_{0}\,\pi }\right)$
      | Automatically generated on 2025-10-31 19:34:32 .
  State_psi_1d_SG_D_1_de078 : Inport
  State_psi_d_SG_D_1_bbc2d : Inport  Port=2
  State_psi_fd_SG_D_1_530eb : Inport  Port=3
  Input_v_d_SG_D_1_cbb22 : Inport  Port=4
  State_theta_SG_D_1_f5fac : Inport  Port=5
  Input_v_q_SG_D_1_0bc0c : Inport  Port=6
  State_theta_SG_D_1_d58f8 : Inport  Port=7
  State_psi_q_SG_D_1_b67fc : Inport  Port=8
  State_w_SG_D_1_d7dd0 : Inport  Port=9
  Add_2708b : Sum
  Add_657c5 : Sum
  Constant_-1_8777e : Constant  Value=-1
  Constant_-2.0_74d9a : Constant  Value=-2.0
  Constant_2.0_81462 : Constant  Value=2.0
  Constant_R_a_b55a6 : Constant  Value=R_a
  Constant_f0_3d2b1 : Constant  Value=f0
  Constant_f0_ba6c0 : Constant  Value=f0
  Constant_pi_2c277 : Constant  Value=pi
  Constant_pi_3714a : Constant  Value=pi
  Constant_x_dd_76149 : Constant  Value=x_dd
  Constant_x_dd_9ffaf : Constant  Value=x_dd
  Constant_x_dd_ba02f : Constant  Value=x_dd
  Constant_x_ddd_d998b : Constant  Value=x_ddd
  Constant_x_ddd_e9bf8 : Constant  Value=x_ddd
  Constant_x_ddd_f4e93 : Constant  Value=x_ddd
  Constant_x_l_6953c : Constant  Value=x_l
  Constant_x_l_ca12d : Constant  Value=x_l
  Constant_x_l_e5e0c : Constant  Value=x_l
  Divide_16f5c : Product  Inputs=*/
  Divide_2cd0a : Product  Inputs=*/
  Divide_3e42b : Product  Inputs=*/
  Divide_6d73e : Product  Inputs=*/
  MathFunc_cos_a4407 : Trigonometry  Operator=cos
  MathFunc_sin_4e479 : Trigonometry
  Product_18ef5 : Product
  Product_272b5 : Product
  Product_2b15f : Product
  Product_39cf9 : Product
  Product_44a22 : Product
  Product_48254 : Product
  Product_56873 : Product
  Product_783a8 : Product
  Product_a4ce1 : Product
  Product_a60a2 : Product
  Product_e5d7c : Product
  Product_fb716 : Product
  Subtract_0d296 : Sum  Inputs=+-
  Subtract_48b16 : Sum  Inputs=+-
  Subtract_53dbb : Sum  Inputs=+-
  Subtract_ae264 : Sum  Inputs=+-
  Subtract_aedfd : Sum  Inputs=+-
  Subtract_b0c8f : Sum  Inputs=+-
  Subtract_eeeda : Sum  Inputs=+-
  Blockout_d_psi_d_SG_D_1_d98e5 : Outport
  wires:
  Add_657c5/1 -> Subtract_b0c8f/1
  Product_48254/1 -> Divide_16f5c/1
  Subtract_48b16/1 -> Product_48254/2
  Divide_16f5c/1 -> Add_657c5/1
  Product_fb716/1 -> Product_48254/1
  Constant_x_ddd_d998b/1 -> Subtract_48b16/2
  Constant_x_dd_76149/1 -> Subtract_48b16/1
  State_psi_1d_SG_D_1_de078/1 -> Product_fb716/2
  Constant_-1_8777e/1 -> Product_fb716/1
  Product_56873/1 -> Divide_6d73e/1
  Constant_x_l_6953c/1 -> Subtract_eeeda/2
  State_psi_d_SG_D_1_bbc2d/1 -> Add_657c5/2
  Constant_x_dd_9ffaf/1 -> Subtract_eeeda/1
  Constant_x_ddd_f4e93/1 -> Subtract_aedfd/1
  Constant_x_l_ca12d/1 -> Subtract_aedfd/2
  Subtract_eeeda/1 -> Divide_16f5c/2
  State_psi_fd_SG_D_1_530eb/1 -> Product_56873/1
  Constant_x_ddd_e9bf8/1 -> Divide_2cd0a/2
  Subtract_aedfd/1 -> Product_56873/2
  Product_18ef5/1 -> Subtract_0d296/2
  Constant_x_dd_ba02f/1 -> Subtract_ae264/1
  Constant_x_l_e5e0c/1 -> Subtract_ae264/2
  Subtract_ae264/1 -> Divide_6d73e/2
  Divide_6d73e/1 -> Subtract_b0c8f/2
  Constant_R_a_b55a6/1 -> Product_a60a2/1
  Subtract_b0c8f/1 -> Product_a60a2/2
  MathFunc_cos_a4407/1 -> Product_44a22/2
  State_theta_SG_D_1_f5fac/1 -> MathFunc_sin_4e479/1
  Divide_2cd0a/1 -> Subtract_0d296/1
  Product_a60a2/1 -> Divide_2cd0a/1
  MathFunc_sin_4e479/1 -> Product_18ef5/2
  Input_v_d_SG_D_1_cbb22/1 -> Product_18ef5/1
  Product_a4ce1/1 -> Blockout_d_psi_d_SG_D_1_d98e5/1
  Product_2b15f/1 -> Product_a4ce1/1
  Product_272b5/1 -> Product_2b15f/1
  State_theta_SG_D_1_d58f8/1 -> MathFunc_cos_a4407/1
  Constant_2.0_81462/1 -> Product_e5d7c/1
  Constant_pi_2c277/1 -> Product_e5d7c/2
  Input_v_q_SG_D_1_0bc0c/1 -> Product_44a22/1
  Constant_f0_3d2b1/1 -> Product_2b15f/2
  State_psi_q_SG_D_1_b67fc/1 -> Product_783a8/1
  State_w_SG_D_1_d7dd0/1 -> Product_783a8/2
  Product_e5d7c/1 -> Product_39cf9/1
  Constant_pi_3714a/1 -> Product_272b5/2
  Constant_f0_ba6c0/1 -> Product_39cf9/2
  Constant_-2.0_74d9a/1 -> Product_272b5/1
  Add_2708b/1 -> Subtract_53dbb/1
  Subtract_0d296/1 -> Add_2708b/1
  Product_44a22/1 -> Add_2708b/2
  Product_783a8/1 -> Divide_3e42b/1
  Product_39cf9/1 -> Divide_3e42b/2
  Divide_3e42b/1 -> Subtract_53dbb/2
  Subtract_53dbb/1 -> Product_a4ce1/2

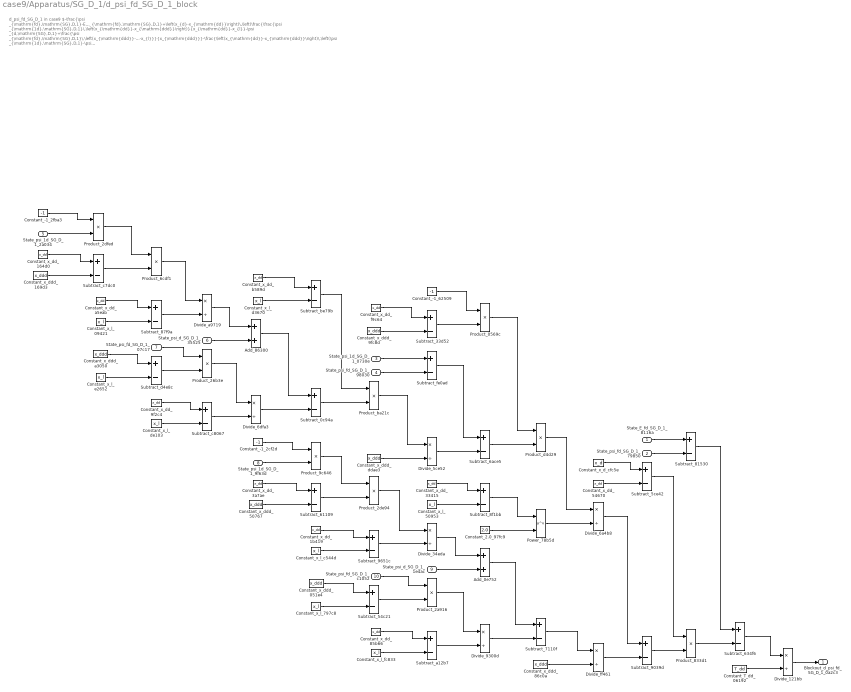
== system case9/Apparatus/SG_D_1/d_psi_fd_SG_D_1_block ==
  note: d_psi_fd_SG_D_1 in case9
      | $-\frac{\psi _{\mathrm{fd},\mathrm{SG},D,1}-E_{\mathrm{fd},\mathrm{SG},D,1}+\left(x_{d}-x_{\mathrm{dd}}\right)\,\left(\frac{\frac{\psi _{\mathrm{1d},\mathrm{SG},D,1}\,\left(x_{\mathrm{dd}}-x_{\mathrm{ddd}}\right)}{x_{\mathrm{dd}}-x_{l}}-\psi _{d,\mathrm{SG},D,1}+\frac{\psi _{\mathrm{fd},\mathrm{SG},D,1}\,\left(x_{\mathrm{ddd}}-x_{l}\right)}{x_{\mathrm{dd}}-x_{l}}}{x_{\mathrm{ddd}}}-\frac{\left(x_{\mathrm{dd}}-x_{\mathrm{ddd}}\right)\,\left(\psi _{\mathrm{1d},\mathrm{SG},D,1}-\psi _{\mathrm{fd},\mathrm{SG},D,1}+\frac{\left(x_{\mathrm{dd}}-x_{l}\right)\,\left(\frac{\psi _{\mathrm{1d},\mathrm{SG},D,1}\,\left(x_{\mathrm{dd}}-x_{\mathrm{ddd}}\right)}{x_{\mathrm{dd}}-x_{l}}-\psi _{d,\mathrm{SG},D,1}+\frac{\psi _{\mathrm{fd},\mathrm{SG},D,1}\,\left(x_{\mathrm{ddd}}-x_{l}\right)}{x_{\mathrm{dd}}-x_{l}}\right)}{x_{\mathrm{ddd}}}\right)}{{\left(x_{\mathrm{dd}}-x_{l}\right)}^2}\right)}{T_{\mathrm{dd}}}$
      | Automatically generated on 2025-10-31 19:34:38 .
  State_E_fd_SG_D_1_8116a : Inport
  State_psi_fd_SG_D_1_79850 : Inport  Port=2
  State_psi_1d_SG_D_1_0730e : Inport  Port=3
  State_psi_fd_SG_D_1_98030 : Inport  Port=4
  State_psi_1d_SG_D_1_2a034 : Inport  Port=5
  State_psi_d_SG_D_1_35525 : Inport  Port=6
  State_psi_fd_SG_D_1_07c17 : Inport  Port=7
  State_psi_1d_SG_D_1_9f63d : Inport  Port=8
  State_psi_d_SG_D_1_1e4ac : Inport  Port=9
  State_psi_fd_SG_D_1_c1052 : Inport  Port=10
  Add_0e752 : Sum
  Add_86300 : Sum
  Constant_-1_2cf2d : Constant  Value=-1
  Constant_-1_2fba3 : Constant  Value=-1
  Constant_-1_62509 : Constant  Value=-1
  Constant_2.0_97fc9 : Constant  Value=2.0
  Constant_T_dd_06192 : Constant  Value=T_dd
  Constant_x_d_cfc5e : Constant  Value=x_d
  Constant_x_dd_164d0 : Constant  Value=x_dd
  Constant_x_dd_1b419 : Constant  Value=x_dd
  Constant_x_dd_33415 : Constant  Value=x_dd
  Constant_x_dd_3a7ae : Constant  Value=x_dd
  Constant_x_dd_54670 : Constant  Value=x_dd
  Constant_x_dd_85b66 : Constant  Value=x_dd
  Constant_x_dd_9f2c4 : Constant  Value=x_dd
  Constant_x_dd_a5eab : Constant  Value=x_dd
  Constant_x_dd_b589d : Constant  Value=x_dd
  Constant_x_dd_f9c64 : Constant  Value=x_dd
  Constant_x_ddd_051e4 : Constant  Value=x_ddd
  Constant_x_ddd_169d3 : Constant  Value=x_ddd
  Constant_x_ddd_50767 : Constant  Value=x_ddd
  Constant_x_ddd_86c0a : Constant  Value=x_ddd
  Constant_x_ddd_9fc8d : Constant  Value=x_ddd
  Constant_x_ddd_a3050 : Constant  Value=x_ddd
  Constant_x_ddd_ddae3 : Constant  Value=x_ddd
  Constant_x_l_09421 : Constant  Value=x_l
  Constant_x_l_50953 : Constant  Value=x_l
  Constant_x_l_797c8 : Constant  Value=x_l
  Constant_x_l_c544d : Constant  Value=x_l
  Constant_x_l_d3670 : Constant  Value=x_l
  Constant_x_l_de103 : Constant  Value=x_l
  Constant_x_l_e2652 : Constant  Value=x_l
  Constant_x_l_fc833 : Constant  Value=x_l
  Divide_121bb : Product  Inputs=*/
  Divide_34eda : Product  Inputs=*/
  Divide_5ce52 : Product  Inputs=*/
  Divide_6a4b8 : Product  Inputs=*/
  Divide_6dfa3 : Product  Inputs=*/
  Divide_9300d : Product  Inputs=*/
  Divide_a9719 : Product  Inputs=*/
  Divide_ff461 : Product  Inputs=*/
  Power_78b5d : Math  Operator=pow
  Product_0569c : Product
  Product_26b3e : Product
  Product_2a916 : Product
  Product_2de94 : Product
  Product_2dfed : Product
  Product_6cdf1 : Product
  Product_833d1 : Product
  Product_9c646 : Product
  Product_ba21c : Product
  Product_d4d29 : Product
  Subtract_0c94a : Sum  Inputs=+-
  Subtract_33d52 : Sum  Inputs=+-
  Subtract_54c21 : Sum  Inputs=+-
  Subtract_5ce42 : Sum  Inputs=+-
  Subtract_61109 : Sum  Inputs=+-
  Subtract_634f6 : Sum  Inputs=+-
  Subtract_6ace5 : Sum  Inputs=+-
  Subtract_7110f : Sum  Inputs=+-
  Subtract_81530 : Sum  Inputs=+-
  Subtract_87f9a : Sum  Inputs=+-
  Subtract_8f1bb : Sum  Inputs=+-
  Subtract_9039d : Sum  Inputs=+-
  Subtract_9651c : Sum  Inputs=+-
  Subtract_a12b7 : Sum  Inputs=+-
  Subtract_be79b : Sum  Inputs=+-
  Subtract_c7dc0 : Sum  Inputs=+-
  Subtract_c8067 : Sum  Inputs=+-
  Subtract_d4e8c : Sum  Inputs=+-
  Subtract_fe0ad : Sum  Inputs=+-
  Blockout_d_psi_fd_SG_D_1_0a2c3 : Outport
  wires:
  State_psi_d_SG_D_1_35525/1 -> Add_86300/2
  Constant_x_dd_a5eab/1 -> Subtract_87f9a/1
  Product_6cdf1/1 -> Divide_a9719/1
  Subtract_c7dc0/1 -> Product_6cdf1/2
  Subtract_0c94a/1 -> Product_ba21c/2
  Product_2dfed/1 -> Product_6cdf1/1
  Constant_x_dd_164d0/1 -> Subtract_c7dc0/1
  Constant_x_l_d3670/1 -> Subtract_be79b/2
  Constant_-1_2fba3/1 -> Product_2dfed/1
  Subtract_be79b/1 -> Product_ba21c/1
  Constant_x_l_09421/1 -> Subtract_87f9a/2
  Constant_x_ddd_169d3/1 -> Subtract_c7dc0/2
  State_psi_1d_SG_D_1_2a034/1 -> Product_2dfed/2
  Constant_x_ddd_a3050/1 -> Subtract_d4e8c/1
  Constant_x_l_e2652/1 -> Subtract_d4e8c/2
  State_E_fd_SG_D_1_8116a/1 -> Subtract_81530/1
  Divide_a9719/1 -> Add_86300/1
  Subtract_87f9a/1 -> Divide_a9719/2
  State_psi_fd_SG_D_1_07c17/1 -> Product_26b3e/1
  Constant_x_ddd_ddae3/1 -> Divide_5ce52/2
  Subtract_d4e8c/1 -> Product_26b3e/2
  Constant_x_dd_9f2c4/1 -> Subtract_c8067/1
  Constant_x_dd_33415/1 -> Subtract_8f1bb/1
  State_psi_fd_SG_D_1_79850/1 -> Subtract_81530/2
  Constant_x_l_de103/1 -> Subtract_c8067/2
  Product_26b3e/1 -> Divide_6dfa3/1
  Constant_-1_62509/1 -> Product_0569c/1
  Subtract_c8067/1 -> Divide_6dfa3/2
  Constant_x_dd_b589d/1 -> Subtract_be79b/1
  Add_86300/1 -> Subtract_0c94a/1
  Constant_x_l_50953/1 -> Subtract_8f1bb/2
  Divide_6dfa3/1 -> Subtract_0c94a/2
  Divide_6a4b8/1 -> Subtract_9039d/1
  Constant_-1_2cf2d/1 -> Product_9c646/1
  State_psi_1d_SG_D_1_9f63d/1 -> Product_9c646/2
  Constant_x_dd_3a7ae/1 -> Subtract_61109/1
  Subtract_33d52/1 -> Product_0569c/2
  Constant_x_ddd_50767/1 -> Subtract_61109/2
  Product_9c646/1 -> Product_2de94/1
  Constant_2.0_97fc9/1 -> Power_78b5d/2
  Product_2de94/1 -> Divide_34eda/1
  Subtract_9039d/1 -> Product_833d1/2
  Subtract_61109/1 -> Product_2de94/2
  State_psi_d_SG_D_1_1e4ac/1 -> Add_0e752/2
  Constant_x_dd_1b419/1 -> Subtract_9651c/1
  Constant_x_l_c544d/1 -> Subtract_9651c/2
  Constant_x_dd_f9c64/1 -> Subtract_33d52/1
  Divide_5ce52/1 -> Subtract_6ace5/2
  Constant_x_ddd_051e4/1 -> Subtract_54c21/1
  Constant_x_ddd_9fc8d/1 -> Subtract_33d52/2
  Constant_x_l_797c8/1 -> Subtract_54c21/2
  Subtract_54c21/1 -> Product_2a916/2
  State_psi_1d_SG_D_1_0730e/1 -> Subtract_fe0ad/1
  Product_2a916/1 -> Divide_9300d/1
  State_psi_fd_SG_D_1_98030/1 -> Subtract_fe0ad/2
  State_psi_fd_SG_D_1_c1052/1 -> Product_2a916/1
  Product_ba21c/1 -> Divide_5ce52/1
  Divide_34eda/1 -> Add_0e752/1
  Subtract_9651c/1 -> Divide_34eda/2
  Constant_x_dd_85b66/1 -> Subtract_a12b7/1
  Constant_x_l_fc833/1 -> Subtract_a12b7/2
  Divide_9300d/1 -> Subtract_7110f/2
  Subtract_fe0ad/1 -> Subtract_6ace5/1
  Subtract_a12b7/1 -> Divide_9300d/2
  Subtract_6ace5/1 -> Product_d4d29/2
  Product_0569c/1 -> Product_d4d29/1
  Subtract_8f1bb/1 -> Power_78b5d/1
  Add_0e752/1 -> Subtract_7110f/1
  Product_d4d29/1 -> Divide_6a4b8/1
  Power_78b5d/1 -> Divide_6a4b8/2
  Subtract_7110f/1 -> Divide_ff461/1
  Constant_x_ddd_86c0a/1 -> Divide_ff461/2
  Constant_x_d_cfc5e/1 -> Subtract_5ce42/1
  Constant_x_dd_54670/1 -> Subtract_5ce42/2
  Divide_ff461/1 -> Subtract_9039d/2
  Subtract_5ce42/1 -> Product_833d1/1
  Subtract_81530/1 -> Subtract_634f6/1
  Product_833d1/1 -> Subtract_634f6/2
  Subtract_634f6/1 -> Divide_121bb/1
  Constant_T_dd_06192/1 -> Divide_121bb/2
  Divide_121bb/1 -> Blockout_d_psi_fd_SG_D_1_0a2c3/1
